simulink model "week3_problem3_2005052"  (R2021a)
settings: Solver=VariableStepAuto  StartTime=0.0  StopTime=10.0  RelTol=1e-3
undefined symbols (not defined in the file): g, I, m, R, v0
settings Model: Creator=admin  LastModifiedBy=admin

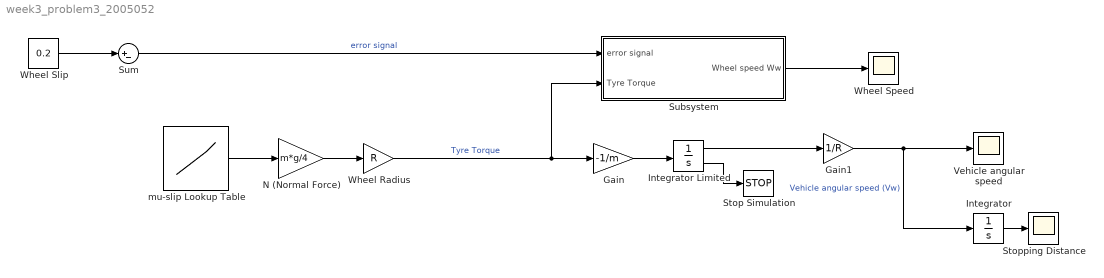
== system week3_problem3_2005052 ==
  Gain : Gain  Gain=-1/m
  Gain1 : Gain  Gain=1/R
  Integrator : Integrator
  Integrator Limited : Integrator  InitialCondition=v0  LimitOutput=on  UpperSaturationLimit=1000  LowerSaturationLimit=0  ShowSaturationPort=on
  N (Normal Force) : Gain  Gain=m*g/4
  Stop Simulation : Stop
  Stopping Distance : Scope
  Subsystem : Subsystem
  Sum : Sum  Inputs=|+-
  Vehicle angular speed : Scope
  Wheel Radius : Gain  Gain=R
  Wheel Slip : Constant  Value=0.2
  Wheel Speed : Scope
  mu-slip Lookup Table : Lookup_n-D  NumberOfTableDimensions=1  BreakpointsForDimension1=[-5:5]  Table=tanh([-5:5])  InternalRulePriority=Speed  RndMeth=Simplest  InputSameDT=on
  wires:
  Wheel Slip/1 -> Sum/1
  mu-slip Lookup Table/1 -> N (Normal Force)/1
  N (Normal Force)/1 -> Wheel Radius/1
  Sum/1 -> Subsystem/1(error signal)  "error signal"
  Wheel Radius/1 -> Gain/1, Subsystem/2(Tyre Torque)  "Tyre Torque"
  Subsystem/1(Wheel speed Ww) -> Wheel Speed/1
  Gain/1 -> Integrator Limited/1
  Integrator Limited/1 -> Gain1/1
  Gain1/1 -> Integrator/1, Vehicle angular speed/1  "Vehicle angular speed (Vw)"
  Integrator Limited/2 -> Stop Simulation/1
  Integrator/1 -> Stopping Distance/1

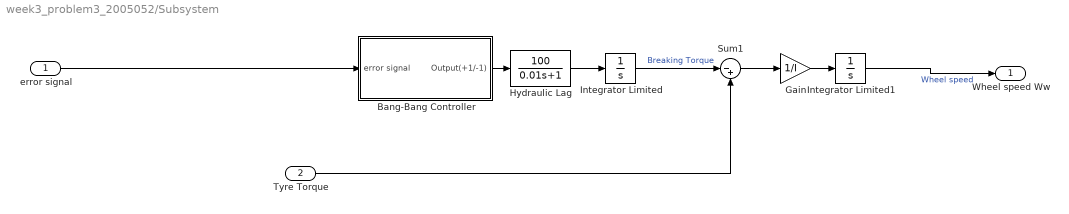
== system week3_problem3_2005052/Subsystem ==
  error signal : Inport
  Tyre Torque : Inport  Port=2
  Bang-Bang Controller : Subsystem
  Gain : Gain  Gain=1/I
  Hydraulic Lag : TransferFcn  Numerator=[100]  Denominator=[0.01 1]
  Integrator Limited : Integrator  LimitOutput=on  UpperSaturationLimit=1000  LowerSaturationLimit=0
  Integrator Limited1 : Integrator  InitialCondition=v0/R  LimitOutput=on  UpperSaturationLimit=1000  LowerSaturationLimit=0
  Sum1 : Sum  Inputs=|-+
  Wheel speed Ww : Outport
  wires:
  Sum1/1 -> Gain/1
  Integrator Limited/1 -> Sum1/1  "Breaking Torque"
  error signal/1 -> Bang-Bang Controller/1(error signal)
  Tyre Torque/1 -> Sum1/2
  Hydraulic Lag/1 -> Integrator Limited/1
  Bang-Bang Controller/1(Output(+1/-1)) -> Hydraulic Lag/1
  Gain/1 -> Integrator Limited1/1
  Integrator Limited1/1 -> Wheel speed Ww/1  "Wheel speed"

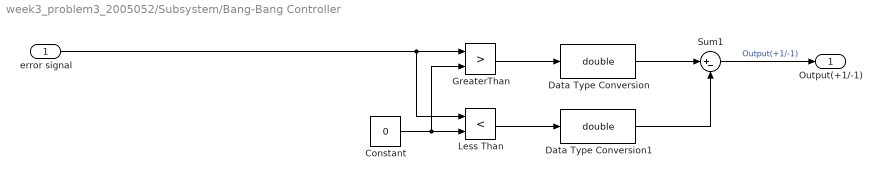
== system week3_problem3_2005052/Subsystem/Bang-Bang Controller ==
  error signal : Inport
  Constant : Constant  Value=0
  Data Type Conversion : DataTypeConversion  OutDataTypeStr=double  RndMeth=Zero
  Data Type Conversion1 : DataTypeConversion  OutDataTypeStr=double  RndMeth=Zero
  GreaterThan : RelationalOperator  Operator=>  OutDataTypeStr=boolean  RndMeth=Simplest
  Less Than : RelationalOperator  Operator=<  OutDataTypeStr=boolean  RndMeth=Simplest
  Sum1 : Sum  Inputs=|+-
  Output(+1/-1) : Outport
  wires:
  GreaterThan/1 -> Data Type Conversion/1
  Sum1/1 -> Output(+1/-1)/1  "Output(+1/-1)"
  Constant/1 -> GreaterThan/2, Less Than/2
  Less Than/1 -> Data Type Conversion1/1
  error signal/1 -> GreaterThan/1, Less Than/1
  Data Type Conversion1/1 -> Sum1/2
  Data Type Conversion/1 -> Sum1/1
